simulink model "RequirementsLogicTest"  (R2024a)
settings: Solver=VariableStepAuto  StartTime=0.0  StopTime=10.0  RelTol=1e-3
settings Model: Creator=david  LastModifiedBy=david

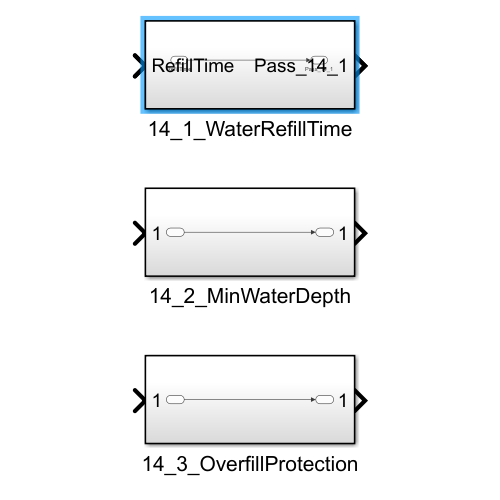
[thumbnail: Simulink's stored preview of the top-level diagram]
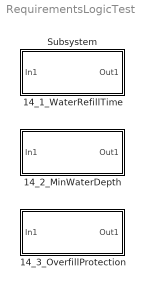
== system RequirementsLogicTest ==
  14_1_WaterRefillTime : Subsystem
  14_2_MinWaterDepth : Subsystem
  14_3_OverfillProtection : Subsystem
  Subsystem : Subsystem

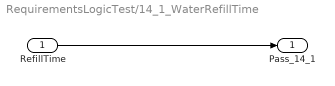
== system RequirementsLogicTest/14_1_WaterRefillTime ==
  RefillTime : Inport
  Pass_14_1 : Outport
  wires:
  RefillTime/1 -> Pass_14_1/1

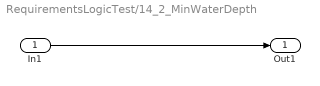
== system RequirementsLogicTest/14_2_MinWaterDepth ==
  In1 : Inport
  Out1 : Outport
  wires:
  In1/1 -> Out1/1

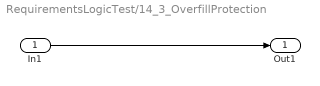
== system RequirementsLogicTest/14_3_OverfillProtection ==
  In1 : Inport
  Out1 : Outport
  wires:
  In1/1 -> Out1/1

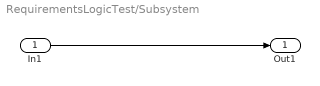
== system RequirementsLogicTest/Subsystem ==
  In1 : Inport
  Out1 : Outport
  wires:
  In1/1 -> Out1/1
